simulink model "flanger_mono_ref"  (R2020b)
settings: Solver=FixedStepDiscrete  StartTime=0.0  StopTime=stopTime  FixedStep=1.0416666666666666e-05  RelTol=1e-3
values from neighbouring files (symbols this model uses):
  mp = sm_init_avalon_signals(mp)    [sm_callback_init.m]
libraries: hdlsllib x3, dspsigops x1
settings Model: Creator=Ross  LastModifiedBy=wickh
settings DataIOCC: SaveOutput=off  SaveTime=off  ReturnWorkspaceOutputs=off
settings OptimizationCC: BlockReduction=off  ConditionallyExecuteInputs=off  DefaultParameterBehavior=Inlined  SimCompilerOptimization=on
settings DebuggingCC: ReadBeforeWriteMsg=DisableAll  WriteAfterWriteMsg=DisableAll  WriteAfterReadMsg=DisableAll  AlgebraicLoopMsg=error  MultiTaskDSMMsg=none  SingleTaskRateTransMsg=error  PregeneratedLibrarySubsystemCodeDiagnostic=none  ArithmeticOperatorsInVariantConditions=warning
settings HardwareCC: ProdBitPerPointer=32  ProdBitPerSizeT=32  ProdBitPerPtrDiffT=32  ProdLargestAtomicFloat=None  ProdIntDivRoundTo=Undefined  ProdEndianess=Unspecified  ProdWordSize=32  ProdHWDeviceType=ASIC/FPGA->ASIC/FPGA  TargetBitPerPointer=64  TargetBitPerSizeT=64  TargetBitPerPtrDiffT=64  TargetLongLongMode=on  TargetIntDivRoundTo=Zero  TargetEndianess=LittleEndian  TargetWordSize=64  TargetHWDeviceType=Custom Processor->MATLAB Host Computer  ProdEqTarget=off
settings ModelReferenceCC: UpdateModelReferenceTargets=IfOutOfDate
settings SFSimCC: SFSimEcho=off  SimUseLocalCustomCode=off  CustomCodeUndefinedFunction=UseInterfaceOnly
settings RTWCC: RTWUseLocalCustomCode=off

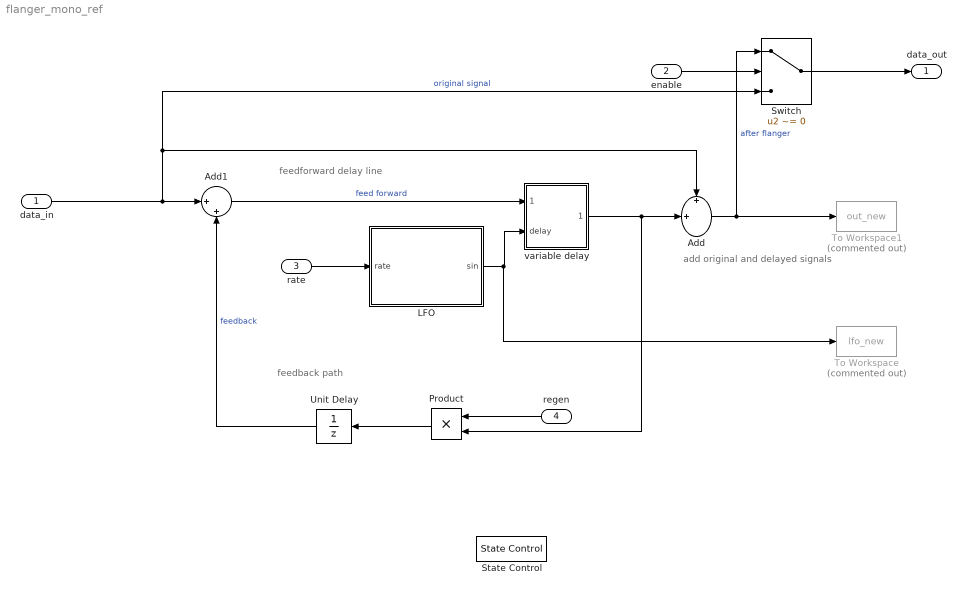
== system flanger_mono_ref ==
  note: add original and delayed signals
  note: feedforward delay line
  note: feedback path
  data_in : Inport  OutDataTypeStr=fixdt(1,24,23)  PortDimensions=1  SampleTime=[1.0416666666666666e-05,0]
  enable : Inport  Port=2  OutDataTypeStr=boolean  PortDimensions=1  SampleTime=[1.0416666666666666e-05,0]
  rate : Inport  Port=3  OutDataTypeStr=fixdt(0,8,5)  PortDimensions=1  SampleTime=[1.0416666666666666e-05,0]
  regen : Inport  Port=4  OutDataTypeStr=fixdt(0,8,7)  PortDimensions=1  SampleTime=[1.0416666666666666e-05,0]
  Add : Sum  Inputs=+|+||  OutDataTypeStr=fixdt(mp.signed, mp.W_bits, mp.F_bits)
  Add1 : Sum  Inputs=||+|+  OutDataTypeStr=fixdt(1, 40, 32)
  LFO : Subsystem
  Product : Product  OutDataTypeStr=Inherit: Inherit via back propagation
  State Control : StateControl  StateControl=Synchronous
  Switch : Switch  Criteria=u2 ~= 0
  To Workspace : ToWorkspace  Commented=on  VariableName=lfo_new  SampleTime=-1
      settings: Save2DSignal=2-D array (concatenate along first dimension)
  To Workspace1 : ToWorkspace  Commented=on  VariableName=out_new  SampleTime=-1
      settings: Save2DSignal=2-D array (concatenate along first dimension)
  Unit Delay : UnitDelay  SampleTime=-1  HasFrameUpgradeWarning=on
  variable delay : Subsystem
  data_out : Outport  OutDataTypeStr=fixdt(1,24,23)  PortDimensions=1  SampleTime=[1.0416666666666666e-05,0]  InitialOutput=0  VectorParamsAs1DForOutWhenUnconnected=off
  wires:
  data_in/1 -> Add/1, Switch/3, Add1/1  "original signal"
  Add/1 -> To Workspace1/1, Switch/1  "after flanger"
  Switch/1 -> data_out/1
  enable/1 -> Switch/2
  rate/1 -> LFO/1(rate)
  regen/1 -> Product/1
  Product/1 -> Unit Delay/1
  Unit Delay/1 -> Add1/2  "feedback"
  variable delay/1(data_out) -> Product/2, Add/2
  Add1/1 -> variable delay/1(data_in)  "feed forward"
  LFO/1(sin) -> variable delay/2(delay), To Workspace/1

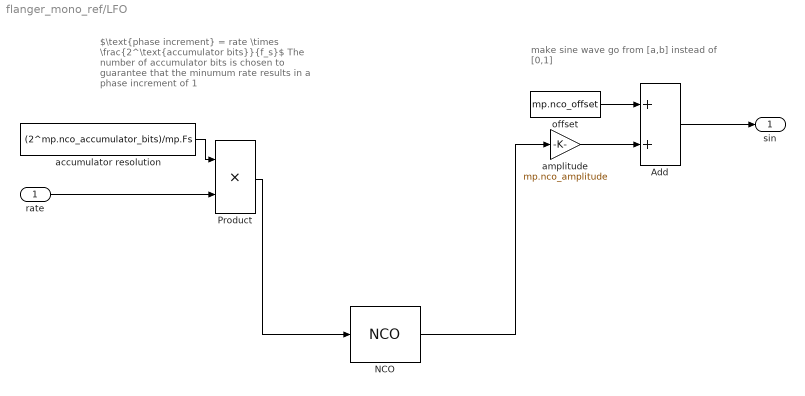
== system flanger_mono_ref/LFO ==
  note: make sine wave go from [a,b]
      | instead of [0,1]
  note: $\text{phase increment} = rate \times \frac{2^\text{accumulator bits}}{f_s}$
      | The number of accumulator bits is chosen to guarantee that the minumum rate results in a phase increment of 1
  rate : Inport
  Add : Sum  OutDataTypeStr=fixdt(0,mp.dpram_addr_size,0)
  NCO : dspsigops/NCO  AccIncSrc=Input port  AccInc=100  PhaseOffsetSrc=Specify via dialog  PhaseOffset=0  AccumWL=16  HasDither=on  DitherWL=mp.nco_dither_bits  PNgeneratorLength=19  HasPhaseQuantizer=on  TableDepth=mp.nco_quantizer_bits  HasOutputPhaseError=off  Formula=Sine  DataType=Binary point scaling  OutputWL=16  OutputFL=14  CompMethod=Table lookup (no interpolation)  SampleTime=1  SamplesPerFrame=1  OutputFrames=off
      settings: SourceProductBaseCode=DS
  Product : Product
  accumulator resolution : Constant  Value=(2^mp.nco_accumulator_bits)/mp.Fs  OutDataTypeStr=fixdt(0,16,12)  SampleTime=-1
  amplitude : Gain  Gain=mp.nco_amplitude  ParamDataTypeStr=uint8
  offset : Constant  Value=mp.nco_offset  OutDataTypeStr=uint8  SampleTime=-1
  sin : Outport  VectorParamsAs1DForOutWhenUnconnected=off
  wires:
  NCO/1 -> amplitude/1
  Add/1 -> sin/1
  offset/1 -> Add/1
  amplitude/1 -> Add/2
  accumulator resolution/1 -> Product/1
  rate/1 -> Product/2
  Product/1 -> NCO/1

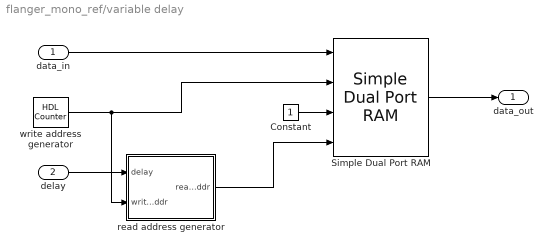
== system flanger_mono_ref/variable delay ==
  data_in : Inport
  delay : Inport  Port=2
  Constant : Constant  OutDataTypeStr=Inherit: Inherit via back propagation  SampleTime=-1
  Simple Dual Port RAM : hdlsllib/HDL RAMs/Simple Dual Port RAM  ram_size=mp.dpram_addr_size
      settings: SourceProductBaseCode=SL
  read address generator : Subsystem
  write address generator : hdlsllib/Sources/HDL Counter  CountType=Count limited  CountInit=0  CountStep=1  CountMax=2^mp.dpram_addr_size - 1  CountFromType=Initial value  CountFrom=0  CountResetPort=off  CountLoadPort=off  CountEnbPort=off  CountDirPort=off  CountDataType=Unsigned  CountWordLen=mp.dpram_addr_size  CountFracLen=0  CountSampTime=-1
  data_out : Outport  VectorParamsAs1DForOutWhenUnconnected=off
  wires:
  delay/1 -> read address generator/1(delay)
  read address generator/1(read_addr) -> Simple Dual Port RAM/4
  data_in/1 -> Simple Dual Port RAM/1
  write address generator/1 -> read address generator/2(write_addr), Simple Dual Port RAM/2
  Simple Dual Port RAM/1 -> data_out/1
  Constant/1 -> Simple Dual Port RAM/3

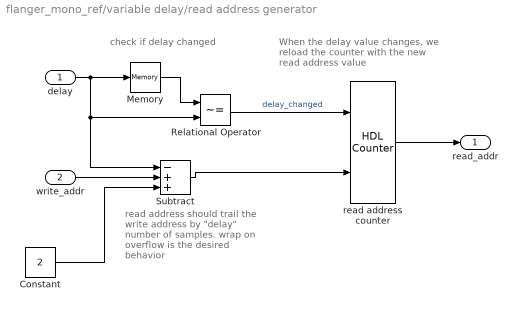
== system flanger_mono_ref/variable delay/read address generator ==
  note: check if delay changed
  note: When the delay value changes, we reload the counter with the new read address value
  note: read address should trail the write address by "delay" number of samples.
      |
      | wrap on overflow is the desired behavior
  delay : Inport
  write_addr : Inport  Port=2
  Constant : Constant  Value=2  OutDataTypeStr=Inherit: Inherit via back propagation  SampleTime=-1
  Memory : Memory  InheritSampleTime=on
  Relational Operator : RelationalOperator  Operator=~=  OutDataTypeStr=boolean  RndMeth=Nearest
  Subtract : Sum  Inputs=-++  InputSameDT=on  OutDataTypeStr=Inherit: Same as first input
  read address counter : hdlsllib/Sources/HDL Counter  CountType=Count limited  CountInit=0  CountStep=1  CountMax=2^mp.dpram_addr_size - 1  CountFromType=Initial value  CountFrom=0  CountResetPort=off  CountLoadPort=on  CountEnbPort=off  CountDirPort=off  CountDataType=Unsigned  CountWordLen=mp.dpram_addr_size  CountFracLen=0  CountSampTime=-1
  read_addr : Outport  VectorParamsAs1DForOutWhenUnconnected=off
  wires:
  Constant/1 -> Subtract/3
  Subtract/1 -> read address counter/2
  write_addr/1 -> Subtract/2
  Relational Operator/1 -> read address counter/1  "delay_changed"
  Memory/1 -> Relational Operator/1
  delay/1 -> Subtract/1, Relational Operator/2, Memory/1
  read address counter/1 -> read_addr/1
